simulink model "sim_instalacja_grzejnikowa"  (R2021b)
settings: Solver=VariableStepAuto  StartTime=0.0  StopTime=160000  MaxStep=5  RelTol=1e-3
undefined symbols (not defined in the file): cpw, Cvcwu, Cvg, Cvk, Cvr, Cvs, Cvw, delay, dfmb, dfmg, dqt, dqtb, dqtb2, dspr, dTset_cwu, dTzew, fmbN, fmgN, Kcg, Kcr, Kcs, Kcw, qk_skok, qtb2N, qtbN, qtN, skok_czas, skok_czas2, Tcwu0, TcwuN, Tgp0, TgpN, Tkz0, TkzN, Trp0, TrpN, Ts0, Tset_cwu, Twew0, TzewN
settings Model: Creator=adams  LastModifiedBy=adams

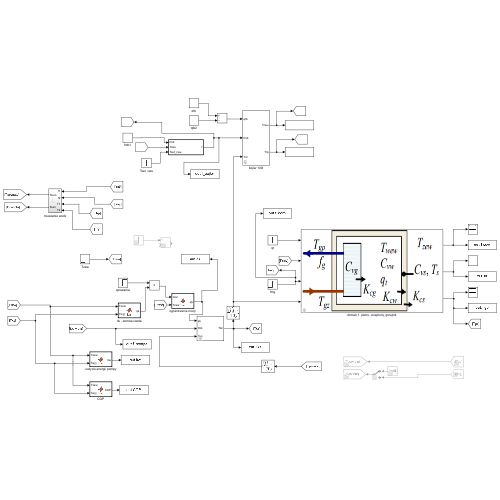
[thumbnail: Simulink's stored preview of the top-level diagram]
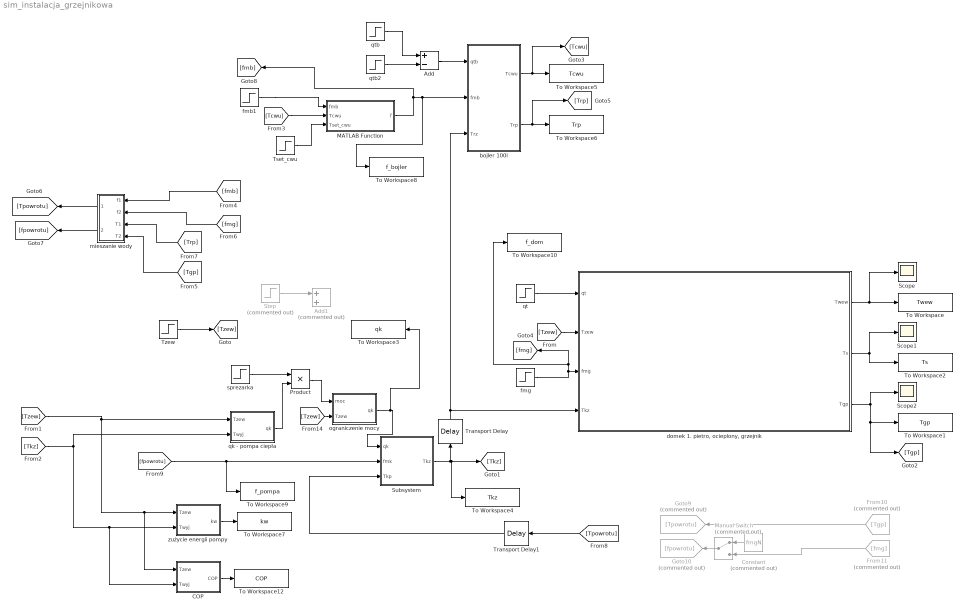
== system sim_instalacja_grzejnikowa ==
  Add : Sum  Inputs=+-
  Add1 : Sum  Commented=on
  COP : MATLAB Function  TreatAsAtomicUnit=on
  Constant : Constant  Commented=on  Value=fmgN
  From10 : From  Commented=on  GotoTag=Tgp
  From11 : From  Commented=on  GotoTag=fmg
  Goto10 : Goto  Commented=on  GotoTag=fpowrotu
  Goto9 : Goto  Commented=on  GotoTag=Tpowrotu
  MATLAB Function : MATLAB Function  TreatAsAtomicUnit=on
  Manual Switch : ManualSwitch  Commented=on
  Product : Product
  Scope : Scope
  Scope1 : Scope
  Scope2 : Scope
  Step : Step  Commented=on  Time=skok_czas  After=qk_skok  SampleTime=0
  Subsystem : Subsystem  mask{Cvk=Cvk, cpw=cpw, Tkz0=Tkz0}
  To Workspace : ToWorkspace  VariableName=Twew  SampleTime=-1
  To Workspace1 : ToWorkspace  VariableName=Tgp  SampleTime=-1
  To Workspace10 : ToWorkspace  VariableName=f_dom  SampleTime=-1
  To Workspace12 : ToWorkspace  VariableName=COP  SampleTime=-1
  To Workspace2 : ToWorkspace  VariableName=Ts  SampleTime=-1
  To Workspace3 : ToWorkspace  VariableName=qk  SampleTime=-1
  To Workspace4 : ToWorkspace  VariableName=Tkz  SampleTime=-1
  To Workspace5 : ToWorkspace  VariableName=Tcwu  SampleTime=-1
  To Workspace6 : ToWorkspace  VariableName=Trp  SampleTime=-1
  To Workspace7 : ToWorkspace  VariableName=kw  SampleTime=-1
  To Workspace8 : ToWorkspace  VariableName=f_bojler  SampleTime=-1
  To Workspace9 : ToWorkspace  VariableName=f_pompa  SampleTime=-1
  Transport Delay : TransportDelay  DelayTime=delay  InitialOutput=TkzN
  Transport Delay1 : TransportDelay  DelayTime=delay  InitialOutput=TgpN
  Tset_cwu : Step  Time=skok_czas  Before=Tset_cwu  After=Tset_cwu+dTset_cwu  SampleTime=0
  Tzew : Step  Time=skok_czas  Before=TzewN  After=TzewN+dTzew  SampleTime=0
  bojler 100l : Subsystem  mask{Kcr=Kcr, cpw=cpw, Cvr=Cvr, Cvcwu=Cvcwu, TcwuN=TcwuN, TrpN=TrpN}
  "domek 1. pietro, ocieplony, grzejnik" : Subsystem  mask{Kcg=Kcg, Cvg=Cvg, Kcw=Kcw, Cvw=Cvw, Kcs=Kcs, Cvs=Cvs, cpw=cpw, Twew0=Twew0, Ts0=Ts0, Tgp0=Tgp0}
      mask Display: image('D:\Dokumenty\Studia\7. sem\praca\obrazki\1.png'); % Use "Edit Image" on toolstrip to change.
  fmb1 : Step  Time=skok_czas  Before=fmbN  After=fmbN+dfmb  SampleTime=0
  fmg : Step  Time=skok_czas  Before=fmgN  After=fmgN+dfmg  SampleTime=0
  mieszanie wody : Subsystem
  ograniczenie mocy : MATLAB Function  TreatAsAtomicUnit=on
  qk - pompa ciepła : MATLAB Function  TreatAsAtomicUnit=on
  qt : Step  Time=skok_czas  Before=qtN  After=qtN+dqt  SampleTime=0
  qtb : Step  Time=skok_czas  Before=qtbN  After=qtbN + dqtb  SampleTime=0
  qtb2 : Step  Time=skok_czas2  Before=qtb2N  After=qtb2N + dqtb2  SampleTime=0  ZeroCross=off
  sprezarka : Step  Time=skok_czas  Before=1  After=1+dspr  SampleTime=0
  zużycie energii pompy : MATLAB Function  TreatAsAtomicUnit=on
  wires:
  [Tzew] -> COP/1(Tzew), zużycie energii pompy/1(Tzew), qk - pompa ciepła/1(Tzew)
  "domek 1. pietro, ocieplony, grzejnik"/2(Ts) -> To Workspace2/1, Scope1/1
  "domek 1. pietro, ocieplony, grzejnik"/1(Twew) -> Scope/1, To Workspace/1
  Transport Delay1/1 -> Subsystem/3(Tkp)
  [Tzew] -> "domek 1. pietro, ocieplony, grzejnik"/2(Tzew)
  Transport Delay/1 -> bojler 100l/3(Trz), "domek 1. pietro, ocieplony, grzejnik"/4(Tkz)
  "domek 1. pietro, ocieplony, grzejnik"/3(Tgp) -> Scope2/1, To Workspace1/1, [Tgp]
  Subsystem/1(Tkz) -> [Tkz], To Workspace4/1, Transport Delay/1
  qk - pompa ciepła/1(qk) -> Product/2
  qtb/1 -> Add/1
  bojler 100l/2(Trp) -> [Trp], To Workspace6/1
  bojler 100l/1(Tcwu) -> [Tcwu], To Workspace5/1
  [Tpowrotu] -> Transport Delay1/1
  qtb2/1 -> Add/2
  Tzew/1 -> [Tzew]
  Add/1 -> bojler 100l/1(qtb)
  qt/1 -> "domek 1. pietro, ocieplony, grzejnik"/1(qt)
  Tset_cwu/1 -> MATLAB Function/3(Tset_cwu)
  [Tcwu] -> MATLAB Function/2(Tcwu)
  fmb1/1 -> MATLAB Function/1(fmb)
  [Tgp] -> mieszanie wody/4(T2)
  [fmg] -> mieszanie wody/2(f2)
  [Trp] -> mieszanie wody/3(T1)
  [fmb] -> mieszanie wody/1(f1)
  mieszanie wody/2(fsum) -> [fpowrotu]
  mieszanie wody/1(Tsum) -> [Tpowrotu]
  From10/1 -> Goto9/1
  Step/1 -> Add1/1
  [Tkz] -> COP/2(Twyj), zużycie energii pompy/2(Twyj), qk - pompa ciepła/2(Twyj)
  [fpowrotu] -> To Workspace9/1, Subsystem/2(fmk)
  MATLAB Function/1(f) -> [fmb], To Workspace8/1, bojler 100l/2(fmb)
  fmg/1 -> To Workspace10/1, [fmg], "domek 1. pietro, ocieplony, grzejnik"/3(fmg)
  From11/1 -> Manual Switch/2
  Constant/1 -> Manual Switch/1
  Manual Switch/1 -> Goto10/1
  Product/1 -> ograniczenie mocy/1(moc)
  sprezarka/1 -> Product/1
  zużycie energii pompy/1(kw) -> To Workspace7/1
  COP/1(COP) -> To Workspace12/1
  [Tzew] -> ograniczenie mocy/2(Tzew)
  ograniczenie mocy/1(qk) -> To Workspace3/1, Subsystem/1(qk)

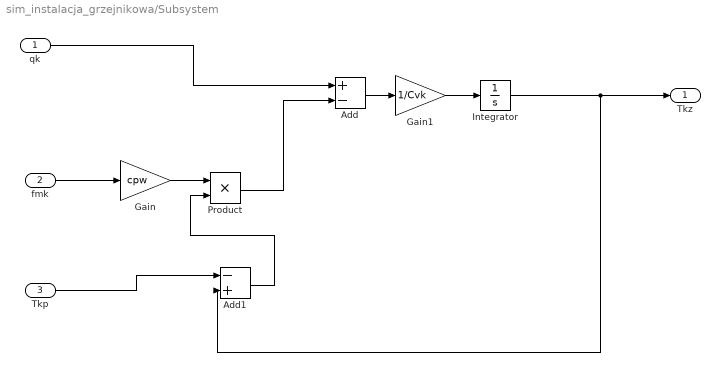
== system sim_instalacja_grzejnikowa/Subsystem ==
  qk : Inport
  fmk : Inport  Port=2
  Tkp : Inport  Port=3
  Add : Sum  Inputs=+-
  Add1 : Sum  Inputs=-+
  Gain : Gain  Gain=cpw
  Gain1 : Gain  Gain=1/Cvk
  Integrator : Integrator  InitialCondition=Tkz0
  Product : Product
  Tkz : Outport
  wires:
  Add1/1 -> Product/2
  Gain/1 -> Product/1
  Integrator/1 -> Add1/2, Tkz/1
  Add/1 -> Gain1/1
  Tkp/1 -> Add1/1
  Gain1/1 -> Integrator/1
  Product/1 -> Add/2
  fmk/1 -> Gain/1
  qk/1 -> Add/1

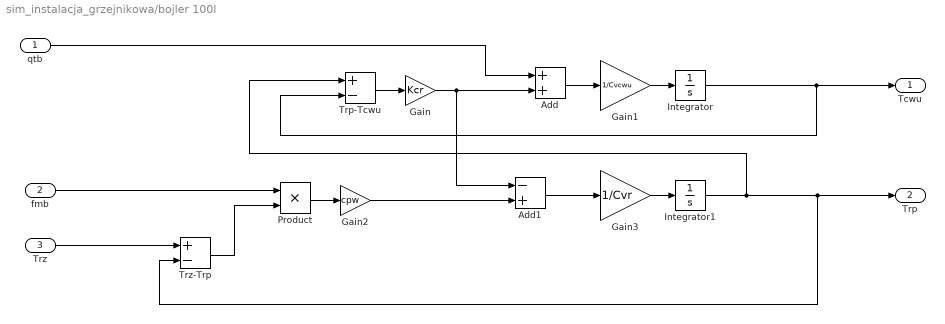
== system sim_instalacja_grzejnikowa/bojler 100l ==
  qtb : Inport
  fmb : Inport  Port=2
  Trz : Inport  Port=3
  Add : Sum
  Add1 : Sum  Inputs=-+
  Gain : Gain  Gain=Kcr
  Gain1 : Gain  Gain=1/Cvcwu
  Gain2 : Gain  Gain=cpw
  Gain3 : Gain  Gain=1/Cvr
  Integrator : Integrator  InitialCondition=Tcwu0
  Integrator1 : Integrator  InitialCondition=Trp0
  Product : Product
  Trp-Tcwu : Sum  Inputs=+-
  Trz-Trp : Sum  Inputs=+-
  Tcwu : Outport
  Trp : Outport  Port=2
  wires:
  Gain/1 -> Add/2, Add1/1
  Add/1 -> Gain1/1
  Trz-Trp/1 -> Product/2
  fmb/1 -> Product/1
  Product/1 -> Gain2/1
  Gain1/1 -> Integrator/1
  Trp-Tcwu/1 -> Gain/1
  Gain3/1 -> Integrator1/1
  Integrator/1 -> Tcwu/1, Trp-Tcwu/2
  Gain2/1 -> Add1/2
  Add1/1 -> Gain3/1
  Integrator1/1 -> Trp-Tcwu/1, Trp/1, Trz-Trp/2
  Trz/1 -> Trz-Trp/1
  qtb/1 -> Add/1

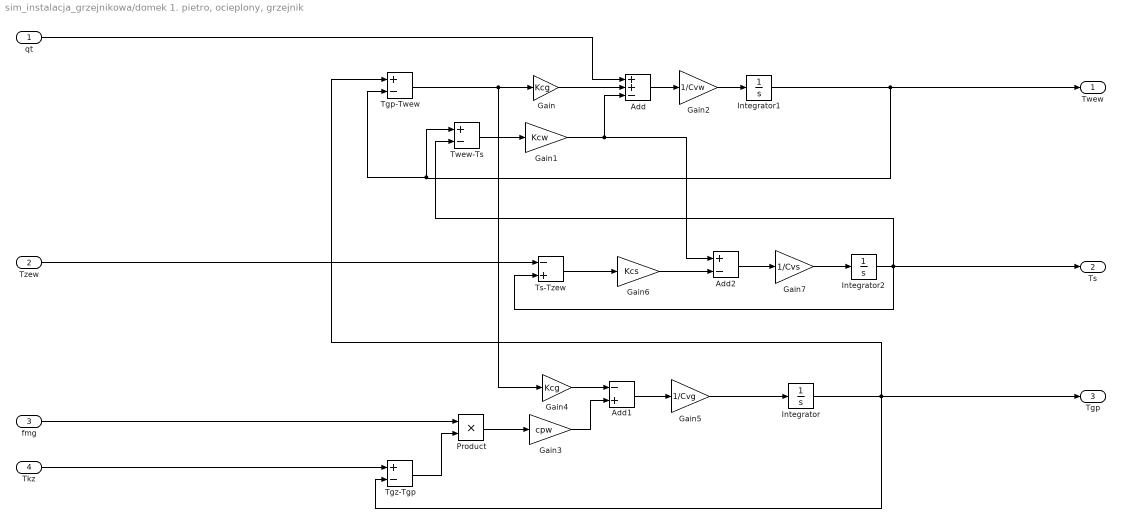
== system sim_instalacja_grzejnikowa/domek 1. pietro, ocieplony, grzejnik ==
  qt : Inport
  Tzew : Inport  Port=2
  fmg : Inport  Port=3
  Tkz : Inport  Port=4
  Add : Sum  Inputs=++-
  Add1 : Sum  Inputs=-+
  Add2 : Sum  Inputs=+-
  Gain : Gain  Gain=Kcg
  Gain1 : Gain  Gain=Kcw
  Gain2 : Gain  Gain=1/Cvw
  Gain3 : Gain  Gain=cpw
  Gain4 : Gain  Gain=Kcg
  Gain5 : Gain  Gain=1/Cvg
  Gain6 : Gain  Gain=Kcs
  Gain7 : Gain  Gain=1/Cvs
  Integrator : Integrator  InitialCondition=Tgp0
  Integrator1 : Integrator  InitialCondition=Twew0
  Integrator2 : Integrator  InitialCondition=Ts0
  Product : Product
  Tgp-Twew : Sum  Inputs=+-
  Tgz-Tgp : Sum  Inputs=+-
  Ts-Tzew : Sum  Inputs=-+
  Twew-Ts : Sum  Inputs=+-
  Twew : Outport
  Ts : Outport  Port=2
  Tgp : Outport  Port=3
  wires:
  Gain1/1 -> Add2/1, Add/3
  Tgp-Twew/1 -> Gain/1, Gain4/1
  Twew-Ts/1 -> Gain1/1
  Gain4/1 -> Add1/1
  Integrator2/1 -> Ts/1, Twew-Ts/2, Ts-Tzew/2
  Gain6/1 -> Add2/2
  qt/1 -> Add/1
  Product/1 -> Gain3/1
  Add/1 -> Gain2/1
  Tgz-Tgp/1 -> Product/2
  Gain7/1 -> Integrator2/1
  Add1/1 -> Gain5/1
  Add2/1 -> Gain7/1
  Integrator1/1 -> Twew/1, Tgp-Twew/2, Twew-Ts/1
  Gain2/1 -> Integrator1/1
  Integrator/1 -> Tgp/1, Tgz-Tgp/2, Tgp-Twew/1
  Ts-Tzew/1 -> Gain6/1
  Gain5/1 -> Integrator/1
  Gain/1 -> Add/2
  Gain3/1 -> Add1/2
  fmg/1 -> Product/1
  Tzew/1 -> Ts-Tzew/1
  Tkz/1 -> Tgz-Tgp/1

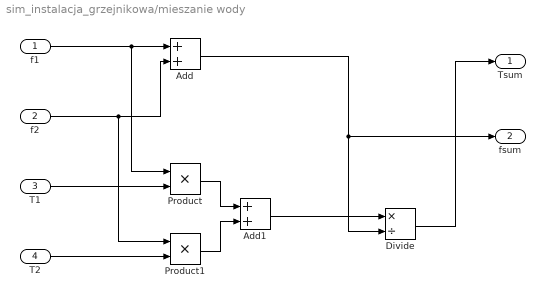
== system sim_instalacja_grzejnikowa/mieszanie wody ==
  f1 : Inport
  f2 : Inport  Port=2
  T1 : Inport  Port=3
  T2 : Inport  Port=4
  Add : Sum
  Add1 : Sum
  Divide : Product  Inputs=*/
  Product : Product
  Product1 : Product
  Tsum : Outport
  fsum : Outport  Port=2
  wires:
  f2/1 -> Add/2, Product1/1
  f1/1 -> Product/1, Add/1
  Add/1 -> fsum/1, Divide/2
  Product1/1 -> Add1/2
  T2/1 -> Product1/2
  Product/1 -> Add1/1
  Add1/1 -> Divide/1
  T1/1 -> Product/2
  Divide/1 -> Tsum/1

== matlab function sim_instalacja_grzejnikowa/qk - pompa ciepła ==
  data: Tzew input; qk output; Twyj input
function qk = fcn(Tzew, Twyj)
qk = 0;
if Twyj >= 50
    if -15 <=Tzew && Tzew < -7
        qk = 445*Tzew + 9995;
    elseif -7 <=Tzew && Tzew < 2
        qk = 830/9*Tzew + 67730/9;
    elseif 2 <=Tzew && Tzew < 7
        qk = 392*Tzew + 6926;
    elseif 7 <=Tzew && Tzew < 10
        qk = -130/3*Tzew + 29920/3;
    elseif 10 <=Tzew && Tzew < 20
        qk = 38*Tzew + 9160;
    elseif 20 <=Tzew && Tzew <= 30
        qk = -56*Tzew + 11040;
    else
         fprintf('Error: Tzew out of range [-15;30]\n'); 
    end
elseif Twyj >= 40 && Twyj < 50
%     if -20 <=Tzew && Tzew < -15
%         qk = 256*Tzew + 9750;
%     elseif -15 <=Tzew && Tzew < 7
    if -15 <=Tzew && Tzew < -7
        qk = 120*Tzew + 7710;
    elseif -7 <=Tzew && Tzew < 2
        qk = 340/3*Tzew + 22990/3;
    elseif 2 <=Tzew && Tzew < 7
        qk = 114*Tzew + 7662;
    elseif 7 <=Tzew && Tzew < 10
        qk = 520/3*Tzew + 21740/3;
    elseif 10 <=Tzew && Tzew < 20
        qk = 16*Tzew + 8820;
    elseif 20 <=Tzew && Tzew <= 30
        qk = -113*Tzew + 11400;
    else
%         fprintf('Error: Tzew out of range [-20;30]\n'); 
        fprintf('Error: Tzew out of range [-15;30]\n'); 
    end
    elseif Twyj < 40
%         if -20 <=Tzew && Tzew < -15
%             qk = 262*Tzew + 10220;
%         elseif -15 <=Tzew && Tzew < -7
        if -15 <=Tzew && Tzew < -7
            qk = -145/4*Tzew + 22985/4;
        elseif -7 <=Tzew && Tzew < 2
            qk = 6000;
        elseif 2 <=Tzew && Tzew < 7
            qk = 426*Tzew + 5148;
        elseif 7 <=Tzew && Tzew < 10
            qk = -190/3*Tzew + 25720/3;
        elseif 10 <=Tzew && Tzew < 20
            qk = 34*Tzew + 7600;
        elseif 20 <=Tzew && Tzew <= 30
            qk = 163*Tzew + 5020;
        else
%             fprintf('Error: Tzew out of range [-20;30]\n'); 
            fprintf('Error: Tzew out of range [-15;30]\n'); 
        end
end

== matlab function sim_instalacja_grzejnikowa/MATLAB Function ==
  data: fmb input; f output; Tcwu input; Tset_cwu input
function f = fcn(fmb, Tcwu, Tset_cwu)
f=fmb;
if Tcwu < Tset_cwu
  f=fmb;
elseif Tcwu >= Tset_cwu
  f=0;
end

== matlab function sim_instalacja_grzejnikowa/COP ==
  data: Tzew input; COP output; Twyj input
function COP = fcn(Tzew, Twyj)
COP = 0;
if Twyj >= 50
    if -15 <=Tzew && Tzew < -7
        COP = 0.105*Tzew + 2.465;
    elseif -7 <=Tzew && Tzew < 2
        COP = 0.0233*Tzew + 1.89333;
    elseif 2 <=Tzew && Tzew < 7
        COP = 0.148*Tzew + 1.644;
    elseif 7 <=Tzew && Tzew < 10
        COP = 0.05*Tzew + 2.33;
    elseif 10 <=Tzew && Tzew < 20
        COP = 0.006*Tzew + 2.77;
    elseif 20 <=Tzew && Tzew <= 30
        COP = 0.042*Tzew + 2.05;
    else
         fprintf('Error: Tzew out of range [-15;30]\n'); 
    end
elseif Twyj >= 40 && Twyj < 50
%     if -20 <=Tzew && Tzew < -15
%         COP = 0.052*Tzew + 2.62;
%     elseif -15 <=Tzew && Tzew < 7
    if -15 <=Tzew && Tzew < -7
        COP = 0.055*Tzew + 2.665;
    elseif -7 <=Tzew && Tzew < 2
        COP = 0.1*Tzew + 2.98;
    elseif 2 <=Tzew && Tzew < 7
        COP = 0.046*Tzew + 3.088;
    elseif 7 <=Tzew && Tzew < 10
        COP = 0.07*Tzew + 2.92;
    elseif 10 <=Tzew && Tzew < 20
        COP = 0.061*Tzew + 3.01;
    elseif 20 <=Tzew && Tzew <= 30
        COP = 0.051*Tzew + 3.21;
    else
%         fprintf('Error: Tzew out of range [-20;30]\n'); 
        fprintf('Error: Tzew out of range [-15;30]\n'); 
    end
    elseif Twyj < 40
%         if -20 <=Tzew && Tzew < -15
%             COP = 0.064*Tzew + 3.18;
%         elseif -15 <=Tzew && Tzew < -7
        if -15 <=Tzew && Tzew < -7
            COP = 0.06*Tzew + 3.12;
        elseif -7 <=Tzew && Tzew < 2
            COP = 0.1*Tzew + 3.4;
        elseif 2 <=Tzew && Tzew < 7
            COP = 0.212*Tzew + 3.176;
        elseif 7 <=Tzew && Tzew < 10
            COP = 0.11*Tzew + 3.89;
        elseif 10 <=Tzew && Tzew < 20
            COP = 0.158*Tzew + 3.41;
        elseif 20 <=Tzew && Tzew <= 30
            COP = -0.058*Tzew + 7.73;
        else
%             fprintf('Error: Tzew out of range [-20;30]\n'); 
            fprintf('Error: Tzew out of range [-15;30]\n'); 
        end
end

== matlab function sim_instalacja_grzejnikowa/ograniczenie mocy ==
  data: moc input; qk output; Tzew input
function qk = fcn(moc, Tzew)
qk = moc;
if Tzew < -2 
    % wg EN 14511 (A–7/W35)
    if moc < 2700
        qk = 2700;
    elseif moc > 7500
        qk = 7500;
    else
        qk = moc;
    end
elseif Tzew >= -2 && Tzew <= 5
    % wg EN 14511 (A2/W35)
    if moc < 3600
        qk = 3600;
    elseif moc > 9000
        qk = 9000;
    else
        qk = moc;
    end
else
    % wg EN 14511 (A7/W35)
    if moc < 4700
        qk = 4700;
    elseif moc > 12000
        qk = 12000;
    else
        qk = moc;
    end
end

== matlab function sim_instalacja_grzejnikowa/zużycie energii pompy ==
  data: Tzew input; kw output; Twyj input
function kw = fcn(Tzew, Twyj)
kw = 0;
if Twyj >= 50
    if -15 <=Tzew && Tzew < -7
        kw = 35*Tzew + 4235;
    elseif -7 <=Tzew && Tzew < 2
        kw = -20/9*Tzew + 35770/9;
    elseif 2 <=Tzew && Tzew < 7
        kw = -72*Tzew + 4114;
    elseif 7 <=Tzew && Tzew < 10
        kw = -80*Tzew + 4170;
    elseif 10 <=Tzew && Tzew < 20
        kw = 6*Tzew + 3310;
    elseif 20 <=Tzew && Tzew <= 30
        kw = -60*Tzew + 4630;
    else
         fprintf('Error: Tzew out of range [-15;30]\n'); 
    end
elseif Twyj >= 40 && Twyj < 50
%     if -20 <=Tzew && Tzew < -15
%         kw = 54*Tzew + 4020;
%     elseif -15 <=Tzew && Tzew < -7
    if -15 <=Tzew && Tzew < -7
        kw = -25*Tzew + 2835;
    elseif -7 <=Tzew && Tzew < 2
        kw = -530/9*Tzew + 23380/9;
    elseif 2 <=Tzew && Tzew < 10
        kw = 2480;
    elseif 10 <=Tzew && Tzew < 20
        kw = -32*Tzew + 2800;
    elseif 20 <=Tzew && Tzew <= 30
        kw = -49*Tzew + 3100;
    else
%         fprintf('Error: Tzew out of range [-20;30]\n'); 
        fprintf('Error: Tzew out of range [-15;30]\n'); 
    end
elseif Twyj < 40
%         if -20 <=Tzew && Tzew < -15
%             kw = 42*Tzew + 3460;
%         elseif -15 <=Tzew && Tzew < -7
    if -15 <=Tzew && Tzew < -7
        kw = -305/4*Tzew + 6745/4;
    elseif -7 <=Tzew && Tzew < 2
        kw = -550/9*Tzew + 16130/9;
    elseif 2 <=Tzew && Tzew < 7
        kw = 14*Tzew + 1642;
    elseif 7 <=Tzew && Tzew < 10
        kw = -170/3*Tzew + 6410/3;
    elseif 10 <=Tzew && Tzew < 20
        kw = -31*Tzew + 1880;
    elseif 20 <=Tzew && Tzew <= 30
        kw = 40*Tzew + 460;
    else
%             fprintf('Error: Tzew out of range [-20;30]\n'); 
        fprintf('Error: Tzew out of range [-15;30]\n'); 
    end
end
